simulink model "updated_target_driver_2026_withVariants"  (R2024b)
settings: Solver=FixedStepDiscrete  StartTime=0.0  StopTime=running_time  FixedStep=dt_s  RelTol=1e-3
values from neighbouring files (symbols this model uses):
  A = gamma_2*gamma_3*Thrust_desired    [force2voltage.m]
  a2_lb = -0.25    [target_driver_setup_2022_Ctrl_V_2_4.m]    (also in target_driver_setup_2022_Ctrl_V_2_4_geometric.m; target_driver_setup_mpc_12msdelay.m; target_driver_setup_mpc_andWLQP.m)
  a2_openloop = -0    (= 0)    [target_driver_setup_2022_Ctrl_V_2_4.m]    (also in target_driver_setup_2022_Ctrl_V_2_4_geometric.m = 0.6; target_driver_setup_mpc_12msdelay.m; target_driver_setup_mpc_andWLQP.m)
  a2_ub = 0.25    [target_driver_setup_2022_Ctrl_V_2_4.m]    (also in target_driver_setup_2022_Ctrl_V_2_4_geometric.m; target_driver_setup_mpc_12msdelay.m; target_driver_setup_mpc_andWLQP.m)
  adaptive_flag = 0    [target_driver_setup_2022_Ctrl_V_2_4.m]    (also in target_driver_setup_2022_Ctrl_V_2_4_geometric.m; target_driver_setup_mpc_12msdelay.m = 1; target_driver_setup_mpc_andWLQP.m = 1)
  adaptive_gain = [gamma_adaptive, adaptive_roll_limit, adaptive_pitch_limit, adaptive_yaw_limit, c_2_adaptive, gamma_lateral_adaptive, adaptive_x_limit, adaptive_y_limit, adaptive_z_limit, c_1_adaptive]    [target_driver_setup_2022_Ctrl_V_2_4.m]    (also in target_driver_setup_2022_Ctrl_V_2_4_geometric.m; target_driver_setup_mpc_12msdelay.m; target_driver_setup_mpc_andWLQP.m)
  adaptive_lateral_flag = 0    [target_driver_setup_2022_Ctrl_V_2_4.m]    (also in target_driver_setup_2022_Ctrl_V_2_4_geometric.m; target_driver_setup_mpc_12msdelay.m = 1; target_driver_setup_mpc_andWLQP.m = 1)
  adaptive_pitch_init = 0    [target_driver_setup_2022_Ctrl_V_2_4.m]    (also in target_driver_setup_2022_Ctrl_V_2_4_geometric.m; target_driver_setup_mpc_12msdelay.m; target_driver_setup_mpc_andWLQP.m)
  adaptive_pitch_limit = 0.1/(scale^2)    (= 1e-07)    [target_driver_setup_2022_Ctrl_V_2_4.m]    (also in target_driver_setup_2022_Ctrl_V_2_4_geometric.m = 3e-07; target_driver_setup_mpc_12msdelay.m; target_driver_setup_mpc_andWLQP.m)
  adaptive_pitch_limit_low = -adaptive_pitch_limit    (= -1e-07)    [target_driver_setup_2022_Ctrl_V_2_4.m]    (also in target_driver_setup_2022_Ctrl_V_2_4_geometric.m = -3e-07; target_driver_setup_mpc_12msdelay.m; target_driver_setup_mpc_andWLQP.m)
  adaptive_roll_init = 0    [target_driver_setup_2022_Ctrl_V_2_4.m]    (also in target_driver_setup_2022_Ctrl_V_2_4_geometric.m; target_driver_setup_mpc_12msdelay.m; target_driver_setup_mpc_andWLQP.m)
  adaptive_roll_limit = 0.3/(scale^2)    (= 3e-07)    [target_driver_setup_2022_Ctrl_V_2_4.m]    (also in target_driver_setup_2022_Ctrl_V_2_4_geometric.m; target_driver_setup_mpc_12msdelay.m; target_driver_setup_mpc_andWLQP.m)
  adaptive_roll_limit_low = -adaptive_roll_limit    (= -3e-07)    [target_driver_setup_2022_Ctrl_V_2_4.m]    (also in target_driver_setup_2022_Ctrl_V_2_4_geometric.m; target_driver_setup_mpc_12msdelay.m; target_driver_setup_mpc_andWLQP.m)
  adaptive_x_init = 0    [target_driver_setup_2022_Ctrl_V_2_4.m]    (also in target_driver_setup_2022_Ctrl_V_2_4_geometric.m; target_driver_setup_mpc_12msdelay.m; target_driver_setup_mpc_andWLQP.m)
  adaptive_x_limit = 0.15/(scale)    (= 0.00015)    [target_driver_setup_2022_Ctrl_V_2_4.m]    (also in target_driver_setup_2022_Ctrl_V_2_4_geometric.m = 7.5e-05; target_driver_setup_mpc_12msdelay.m; target_driver_setup_mpc_andWLQP.m)
  adaptive_x_limit_low = -adaptive_x_limit    (= -0.00015)    [target_driver_setup_2022_Ctrl_V_2_4.m]    (also in target_driver_setup_2022_Ctrl_V_2_4_geometric.m = -7.5e-05; target_driver_setup_mpc_12msdelay.m; target_driver_setup_mpc_andWLQP.m)
  adaptive_y_init = 0    [target_driver_setup_2022_Ctrl_V_2_4.m]    (also in target_driver_setup_2022_Ctrl_V_2_4_geometric.m; target_driver_setup_mpc_12msdelay.m; target_driver_setup_mpc_andWLQP.m)
  adaptive_y_limit = 0.15/(scale)    (= 0.00015)    [target_driver_setup_2022_Ctrl_V_2_4.m]    (also in target_driver_setup_2022_Ctrl_V_2_4_geometric.m = 7.5e-05; target_driver_setup_mpc_12msdelay.m; target_driver_setup_mpc_andWLQP.m)
  adaptive_y_limit_low = -adaptive_y_limit    (= -0.00015)    [target_driver_setup_2022_Ctrl_V_2_4.m]    (also in target_driver_setup_2022_Ctrl_V_2_4_geometric.m = -7.5e-05; target_driver_setup_mpc_12msdelay.m; target_driver_setup_mpc_andWLQP.m)
  adaptive_yaw_init = 0    [target_driver_setup_2022_Ctrl_V_2_4.m]    (also in target_driver_setup_2022_Ctrl_V_2_4_geometric.m; target_driver_setup_mpc_12msdelay.m; target_driver_setup_mpc_andWLQP.m)
  adaptive_yaw_limit = 0.035/(scale^2)    (= 3.5e-08)    [target_driver_setup_2022_Ctrl_V_2_4.m]    (also in target_driver_setup_2022_Ctrl_V_2_4_geometric.m; target_driver_setup_mpc_12msdelay.m; target_driver_setup_mpc_andWLQP.m)
  adaptive_yaw_limit_low = -adaptive_yaw_limit    (= -3.5e-08)    [target_driver_setup_2022_Ctrl_V_2_4.m]    (also in target_driver_setup_2022_Ctrl_V_2_4_geometric.m; target_driver_setup_mpc_12msdelay.m; target_driver_setup_mpc_andWLQP.m)
  adaptive_z_init = 0/scale    (= 0)    [target_driver_setup_2022_Ctrl_V_2_4.m]    (also in target_driver_setup_2022_Ctrl_V_2_4_geometric.m; target_driver_setup_mpc_12msdelay.m; target_driver_setup_mpc_andWLQP.m)
  adaptive_z_limit = 0.20/(scale)    (= 0.0002)    [target_driver_setup_2022_Ctrl_V_2_4.m]    (also in target_driver_setup_2022_Ctrl_V_2_4_geometric.m = 0.0008; target_driver_setup_mpc_12msdelay.m = 0.0008; target_driver_setup_mpc_andWLQP.m = 0.0008)
  adaptive_z_limit_low = -adaptive_z_limit/1    (= -0.0002)    [target_driver_setup_2022_Ctrl_V_2_4.m]    (also in target_driver_setup_2022_Ctrl_V_2_4_geometric.m = -0.0008; target_driver_setup_mpc_12msdelay.m = -0.0008; target_driver_setup_mpc_andWLQP.m = -0.0008)
  att_s = 500    [target_driver_setup_2022_Ctrl_V_2_4.m]    (also in target_driver_setup_2022_Ctrl_V_2_4_geometric.m; target_driver_setup_mpc_12msdelay.m; target_driver_setup_mpc_andWLQP.m)
  b_1_d_desired = [1,0,0]    [target_driver_setup_2022_Ctrl_V_2_4.m]    (also in target_driver_setup_2022_Ctrl_V_2_4_geometric.m; target_driver_setup_mpc_12msdelay.m; target_driver_setup_mpc_andWLQP.m)
  closedloop_flag = 1    [target_driver_setup_2022_Ctrl_V_2_4.m]    (also in target_driver_setup_2022_Ctrl_V_2_4_geometric.m = 0; target_driver_setup_mpc_12msdelay.m = 0; target_driver_setup_mpc_andWLQP.m = 0)
  control_gain = [k_x,k_v, k_R, k_Omega, k_z, k_vz, k_Rx]    [target_driver_setup_2022_Ctrl_V_2_4.m]    (also in target_driver_setup_2022_Ctrl_V_2_4_geometric.m = [k_x,k_v,k_R,k_Omega_pitch,k_Omega_roll,k_z,k_vz,k_Rx]; target_driver_setup_mpc_12msdelay.m = [k_x, k_v, k_R, k_Omega, k_z, k_vz, k_Rx,                  k; target_driver_setup_mpc_andWLQP.m = [k_x, k_v, k_R, k_Omega, k_z, k_vz, k_Rx,                  k)
  delay = delay-vicon_sample_cycle/2    [target_driver_setup_2022_Ctrl_V_2_4.m]    (also in target_driver_setup_2022_Ctrl_V_2_4_geometric.m; target_driver_setup_mpc_12msdelay.m; target_driver_setup_mpc_andWLQP.m)
  drv_amp = abs((vleft_p2p-vright_p2p))/2+min(vleft_p2p,vright_p2p)    [Wing_traj_to_Voltage.m]    (also in force2voltage.m; target_driver_setup_2022_Ctrl_V_2_4.m = 300; target_driver_setup_2022_Ctrl_V_2_4_geometric.m = 110; target_driver_setup_mpc_12msdelay.m = 150)
  drv_bias = max_drv_bias    (= 300)    [target_driver_setup_2022_Ctrl_V_2_4.m]    (also in target_driver_setup_2022_Ctrl_V_2_4_geometric.m = 200; target_driver_setup_mpc_12msdelay.m = 200; target_driver_setup_mpc_andWLQP.m = 200)
  drv_pitch_left = vleft_pitch    [Wing_traj_to_Voltage.m]    (also in force2voltage.m = 0; target_driver_setup_2022_Ctrl_V_2_4.m = 0; target_driver_setup_2022_Ctrl_V_2_4_geometric.m = 9.05; target_driver_setup_mpc_12msdelay.m = 9.05)
  drv_pitch_right = vright_pitch    [Wing_traj_to_Voltage.m]    (also in force2voltage.m = 0; target_driver_setup_2022_Ctrl_V_2_4.m = 0; target_driver_setup_2022_Ctrl_V_2_4_geometric.m = 9.05; target_driver_setup_mpc_12msdelay.m = 9.05)
  drv_roll = (vleft_p2p-vright_p2p)/4    [Wing_traj_to_Voltage.m]    (also in force2voltage.m; target_driver_setup_2022_Ctrl_V_2_4.m = 0; target_driver_setup_2022_Ctrl_V_2_4_geometric.m = -0.001; target_driver_setup_mpc_12msdelay.m = -0.001)
  dt_s = 1e-3    (= 0.001)    [target_driver_setup_2022_Ctrl_V_2_4.m]    (also in target_driver_setup_2022_Ctrl_V_2_4_geometric.m = 0.0002; target_driver_setup_mpc_12msdelay.m = 0.0002; target_driver_setup_mpc_andWLQP.m = 0.0002)
  f_fin = f    (= 180)    [target_driver_setup_2022_Ctrl_V_2_4.m]    (also in target_driver_setup_2022_Ctrl_V_2_4_geometric.m = 155; target_driver_setup_mpc_12msdelay.m = 155; target_driver_setup_mpc_andWLQP.m = 155)
  f_int = f    (= 180)    [target_driver_setup_2022_Ctrl_V_2_4.m]    (also in target_driver_setup_2022_Ctrl_V_2_4_geometric.m = 155; target_driver_setup_mpc_12msdelay.m = 155; target_driver_setup_mpc_andWLQP.m = 155)
  g = 9.8    [target_driver_setup_2022_Ctrl_V_2_4.m]    (also in target_driver_setup_2022_Ctrl_V_2_4_geometric.m; target_driver_setup_mpc_12msdelay.m; target_driver_setup_mpc_andWLQP.m = 9.81; test_full_attitude_mpc.m = 9.81)
  I_moment_vec = [Ixx, Iyy, Izz]    [target_driver_setup_2022_Ctrl_V_2_4.m]    (also in target_driver_setup_2022_Ctrl_V_2_4_geometric.m; target_driver_setup_mpc_12msdelay.m; target_driver_setup_mpc_andWLQP.m)
  landing_flag = 0    [target_driver_setup_2022_Ctrl_V_2_4.m]    (also in target_driver_setup_2022_Ctrl_V_2_4_geometric.m; target_driver_setup_mpc_12msdelay.m; target_driver_setup_mpc_andWLQP.m)
  landing_parameter = [start_delay+T,transition_rate, rising_time, falling_time, landing_rising_time, landing_z_decrease, landing_y_decrease, landing_x_decrease]    [target_driver_setup_2022_Ctrl_V_2_4.m]    (also in target_driver_setup_2022_Ctrl_V_2_4_geometric.m; target_driver_setup_mpc_12msdelay.m; target_driver_setup_mpc_andWLQP.m)
  low_bound = -8    [target_driver_setup_2022_Ctrl_V_2_4.m]    (also in target_driver_setup_2022_Ctrl_V_2_4_geometric.m = -5; target_driver_setup_mpc_12msdelay.m = -10; target_driver_setup_mpc_andWLQP.m = -10)
  low_bound_eR = -0.8    [target_driver_setup_2022_Ctrl_V_2_4.m]    (also in target_driver_setup_2022_Ctrl_V_2_4_geometric.m = -1.2; target_driver_setup_mpc_12msdelay.m = -1.2; target_driver_setup_mpc_andWLQP.m = -1.2)
  low_bound_vx = -0.5    [target_driver_setup_2022_Ctrl_V_2_4.m]    (also in target_driver_setup_2022_Ctrl_V_2_4_geometric.m; target_driver_setup_mpc_12msdelay.m; target_driver_setup_mpc_andWLQP.m)
  low_bound_vy = -0.5    [target_driver_setup_2022_Ctrl_V_2_4.m]    (also in target_driver_setup_2022_Ctrl_V_2_4_geometric.m; target_driver_setup_mpc_12msdelay.m; target_driver_setup_mpc_andWLQP.m)
  low_bound_vz = -0.5    [target_driver_setup_2022_Ctrl_V_2_4.m]    (also in target_driver_setup_2022_Ctrl_V_2_4_geometric.m; target_driver_setup_mpc_12msdelay.m; target_driver_setup_mpc_andWLQP.m)
  low_bound_x = -0.06    [target_driver_setup_2022_Ctrl_V_2_4.m]    (also in target_driver_setup_2022_Ctrl_V_2_4_geometric.m = -0.1; target_driver_setup_mpc_12msdelay.m = -0.6; target_driver_setup_mpc_andWLQP.m = -0.6)
  low_bound_y = -0.06    [target_driver_setup_2022_Ctrl_V_2_4.m]    (also in target_driver_setup_2022_Ctrl_V_2_4_geometric.m; target_driver_setup_mpc_12msdelay.m = -0.6; target_driver_setup_mpc_andWLQP.m = -0.6)
  low_bound_z = -0.04    [target_driver_setup_2022_Ctrl_V_2_4.m]    (also in target_driver_setup_2022_Ctrl_V_2_4_geometric.m; target_driver_setup_mpc_12msdelay.m = -0.1; target_driver_setup_mpc_andWLQP.m = -0.1)
  m = t <= t_zoom    [plot_roll_torque_cmd_vs_actual.m]    (also in plot_roll_torque_cmd_vs_actual_flightlog.m = t >= t0 & t <= t1; target_driver_setup_2022_Ctrl_V_2_4.m = 0.000124; target_driver_setup_2022_Ctrl_V_2_4_geometric.m = 8.5655e-05; target_driver_setup_mpc_12msdelay.m = 8.5655e-05)
  params_vec = [params_opt.delta_1, params_opt.delta_2, params_opt.delta_3,      params_opt.gamma_1, params_opt.gamma_2_1, params_opt.gamma_3,      params_opt.eta, params_opt.nu, params_opt.mu]'    [force2voltage_tuningSandbox.m]    (also in target_driver_setup_2022_Ctrl_V_2_4.m = [params_opt.delta_1, params_opt.delta_2, params_opt.delta_3,; target_driver_setup_2022_Ctrl_V_2_4_geometric.m = [params_opt.delta_1, params_opt.delta_2, params_opt.delta_3,; target_driver_setup_mpc_12msdelay.m = [params_opt.delta_1, params_opt.delta_2, params_opt.delta_3,; target_driver_setup_mpc_andWLQP.m = [params_opt.delta_1, params_opt.delta_2, params_opt.delta_3,)
  phase = 0    [target_driver_setup_2022_Ctrl_V_2_4.m]    (also in target_driver_setup_2022_Ctrl_V_2_4_geometric.m; target_driver_setup_mpc_12msdelay.m; target_driver_setup_mpc_andWLQP.m)
  r_desired = [default_x, default_y,z_desired]    [target_driver_setup_2022_Ctrl_V_2_4.m]    (also in target_driver_setup_2022_Ctrl_V_2_4_geometric.m; target_driver_setup_mpc_12msdelay.m; target_driver_setup_mpc_andWLQP.m)
  roll_offset_angle = 0    [target_driver_setup_2022_Ctrl_V_2_4.m]    (also in target_driver_setup_2022_Ctrl_V_2_4_geometric.m; target_driver_setup_mpc_12msdelay.m; target_driver_setup_mpc_andWLQP.m)
  running_time = start_delay+total_T    (= 9)    [target_driver_setup_2022_Ctrl_V_2_4.m]    (also in target_driver_setup_2022_Ctrl_V_2_4_geometric.m = 10; target_driver_setup_mpc_12msdelay.m = 0.5; target_driver_setup_mpc_andWLQP.m = 10)
  running_time_control = start_delay_control+total_T+0.0    (= 7.1)    [target_driver_setup_2022_Ctrl_V_2_4.m]    (also in target_driver_setup_2022_Ctrl_V_2_4_geometric.m = 10; target_driver_setup_mpc_12msdelay.m = 0.5; target_driver_setup_mpc_andWLQP.m = 10)
  sampling_f = 10000    [target_driver_setup_2022_Ctrl_V_2_4.m]    (also in target_driver_setup_2022_Ctrl_V_2_4_geometric.m = 5000; target_driver_setup_mpc_12msdelay.m = 5000; target_driver_setup_mpc_andWLQP.m = 5000)
  start_delay = 2.0    (= 2)    [target_driver_setup_2022_Ctrl_V_2_4.m]    (also in target_driver_setup_2022_Ctrl_V_2_4_geometric.m = 0; target_driver_setup_mpc_12msdelay.m = 0; target_driver_setup_mpc_andWLQP.m = 0)
  start_delay_control = start_delay + ramp_delay    (= 0.1)    [target_driver_setup_2022_Ctrl_V_2_4.m]    (also in target_driver_setup_2022_Ctrl_V_2_4_geometric.m = 0; target_driver_setup_mpc_12msdelay.m = 0; target_driver_setup_mpc_andWLQP.m = 0)
  T = 1    [target_driver_setup_2022_Ctrl_V_2_4.m]    (also in target_driver_setup_2022_Ctrl_V_2_4_geometric.m = 10; target_driver_setup_mpc_12msdelay.m = 0.5; target_driver_setup_mpc_andWLQP.m = 10; test_full_attitude_mpc.m = T0 + nu(1))
  task_flag = 0    [target_driver_setup_2022_Ctrl_V_2_4.m]    (also in target_driver_setup_2022_Ctrl_V_2_4_geometric.m; target_driver_setup_mpc_12msdelay.m; target_driver_setup_mpc_andWLQP.m)
  task_parameter = [radius_ref, frequency_ref, radius_ratio, lissajous_ratio, lissajous_delta, lissajous_amplitude_ratio,z_radius_ratio]    [target_driver_setup_2022_Ctrl_V_2_4.m]    (also in target_driver_setup_2022_Ctrl_V_2_4_geometric.m; target_driver_setup_mpc_12msdelay.m; target_driver_setup_mpc_andWLQP.m)
  upp_bound = 8    [target_driver_setup_2022_Ctrl_V_2_4.m]    (also in target_driver_setup_2022_Ctrl_V_2_4_geometric.m = 5; target_driver_setup_mpc_12msdelay.m = 10; target_driver_setup_mpc_andWLQP.m = 10)
  upp_bound_eR = 0.8    [target_driver_setup_2022_Ctrl_V_2_4.m]    (also in target_driver_setup_2022_Ctrl_V_2_4_geometric.m = 1.2; target_driver_setup_mpc_12msdelay.m = 1.2; target_driver_setup_mpc_andWLQP.m = 1.2)
  upp_bound_vx = 0.5    [target_driver_setup_2022_Ctrl_V_2_4.m]    (also in target_driver_setup_2022_Ctrl_V_2_4_geometric.m; target_driver_setup_mpc_12msdelay.m; target_driver_setup_mpc_andWLQP.m)
  upp_bound_vy = 0.5    [target_driver_setup_2022_Ctrl_V_2_4.m]    (also in target_driver_setup_2022_Ctrl_V_2_4_geometric.m; target_driver_setup_mpc_12msdelay.m; target_driver_setup_mpc_andWLQP.m)
  upp_bound_vz = 0.5    [target_driver_setup_2022_Ctrl_V_2_4.m]    (also in target_driver_setup_2022_Ctrl_V_2_4_geometric.m; target_driver_setup_mpc_12msdelay.m; target_driver_setup_mpc_andWLQP.m)
  upp_bound_x = 0.06    [target_driver_setup_2022_Ctrl_V_2_4.m]    (also in target_driver_setup_2022_Ctrl_V_2_4_geometric.m = 0.1; target_driver_setup_mpc_12msdelay.m = 0.6; target_driver_setup_mpc_andWLQP.m = 0.6)
  upp_bound_y = 0.06    [target_driver_setup_2022_Ctrl_V_2_4.m]    (also in target_driver_setup_2022_Ctrl_V_2_4_geometric.m; target_driver_setup_mpc_12msdelay.m = 0.6; target_driver_setup_mpc_andWLQP.m = 0.6)
  upp_bound_z = 0.04    [target_driver_setup_2022_Ctrl_V_2_4.m]    (also in target_driver_setup_2022_Ctrl_V_2_4_geometric.m; target_driver_setup_mpc_12msdelay.m = 0.1; target_driver_setup_mpc_andWLQP.m = 0.1)
undefined symbols (not defined in the file or in its folder): Com1, DiscIntNeverNeededParam, dspblkCoreblockFVToolHelper, gcbh, left_mapping, left_mapping_F_to_Phi, lp_den, lp_num, none, right_mapping, right_mapping_F_to_Phi, vlp_den, vlp_num
libraries: simulink x20, xpcseriallib x2, xpcnilib x1, xpcutilitieslib x1
(part 4 of 6)

== system updated_target_driver_2026_withVariants/Vicon Post Processing1/Vicon Validity check/Variant Subsystem1/Simulation ==
  In1 : Inport
  Discrete Pulse Generator : DiscretePulseGenerator  Period=5  SampleTime=dt_s
  Terminator : Terminator
  Out1 : Outport
  wires:
  Discrete Pulse Generator/1 -> Out1/1
  In1/1 -> Terminator/1

== system updated_target_driver_2026_withVariants/Variant Subsystem/Experimental/signal generator a3/Bias_Signal/AveragedBias ==
  note: To avoid having signal "jump",
      | we want SMOOTH transitions
      | in frequency (i.e., a weighted sum
      | of current freq and freq some delta t ago)
  note: time constant = 0.002sec
  In1 : Inport
  Discrete Transfer Fcn : DiscreteTransferFcn  Numerator=[0.05]  Denominator=[1 -.95]
  Out1 : Outport
  wires:
  In1/1 -> Discrete Transfer Fcn/1
  Discrete Transfer Fcn/1 -> Out1/1

== system updated_target_driver_2026_withVariants/Variant Subsystem/Experimental/signal generator a3/Bias_Signal/SIgnalForRamp_binary ==
  note: Should output 1 or -1,
      | so signal ramps UP to 1
      | or DOWN to 0.
  In1 : Inport
  Add : Sum  Inputs=+-
  Compare To Zero : simulink/Logic and Bit Operations/Compare To Zero  relop=>  OutDataTypeStr=uint8  ZeroCross=off
  Constant : Constant
  Data Type Conversion : DataTypeConversion  OutDataTypeStr=double  SaturateOnIntegerOverflow=off  RndMeth=Floor
  Gain : Gain  Gain=2
  Out1 : Outport
  wires:
  In1/1 -> Compare To Zero/1
  Compare To Zero/1 -> Data Type Conversion/1
  Gain/1 -> Add/1
  Constant/1 -> Add/2
  Add/1 -> Out1/1
  Data Type Conversion/1 -> Gain/1

== system updated_target_driver_2026_withVariants/Variant Subsystem/Experimental/signal generator a3/Drive_Signal/AveragedAmp_filtered ==
  note: To avoid having signal "jump",
      | we want SMOOTH transitions
      | in frequency (i.e., a weighted sum
      | of current freq and freq some delta t ago)
  note: time constant 0.002sec
      | for 10kHz samping
  In1 : Inport
  Discrete Transfer Fcn : DiscreteTransferFcn  Numerator=[0.05]  Denominator=[1 -.95]
  Out1 : Outport
  wires:
  In1/1 -> Discrete Transfer Fcn/1
  Discrete Transfer Fcn/1 -> Out1/1

== system updated_target_driver_2026_withVariants/Variant Subsystem/Experimental/signal generator a3/Drive_Signal/AveragedOffset_filtered ==
  note: To avoid having signal "jump",
      | we want SMOOTH transitions
      | in frequency (i.e., a weighted sum
      | of current freq and freq some delta t ago)
  note: c
  note: time constant 0.02sec
      | for 10kHz samping
  In1 : Inport
  Discrete Transfer Fcn : DiscreteTransferFcn  Numerator=[0.05]  Denominator=[1 -.95]
  Out1 : Outport
  wires:
  In1/1 -> Discrete Transfer Fcn/1
  Discrete Transfer Fcn/1 -> Out1/1

== system updated_target_driver_2026_withVariants/Variant Subsystem/Experimental/signal generator a3/Drive_Signal/FlattenedSine1 ==
  freq : Inport
  phase : Inport  Port=2
  a2 : Inport  Port=3
  0.1 : Gain  Gain=0.1
  1.1 : Gain  Gain=1.1
  2f : Gain  Gain=2
  2pi : Gain  Gain=2*pi
  3f : Gain  Gain=3
  Add : Sum  Inputs=+++
  Add1 : Sum
  Amplitude Correction : Subsystem  Commented=on
  AveragedAmp_filtered : Subsystem
  Product : Product
  first harmonic : Trigonometry  OutputSignalType=real
  integrate(omega*t) : DiscreteIntegrator  SampleTime=-1  ICPrevOutput=DiscIntNeverNeededParam  ICPrevScaledInput=DiscIntNeverNeededParam
  second harmonic : Trigonometry  OutputSignalType=real
  third harmonic : Trigonometry  OutputSignalType=real
  split cycle signal : Outport
  wires:
  freq/1 -> 2pi/1
  2pi/1 -> integrate(omega*t)/1
  3f/1 -> third harmonic/1
  first harmonic/1 -> 1.1/1
  third harmonic/1 -> 0.1/1
  1.1/1 -> Add/1
  Add1/1 -> first harmonic/1, 2f/1, 3f/1
  integrate(omega*t)/1 -> Add1/1
  phase/1 -> Add1/2
  2f/1 -> second harmonic/1
  0.1/1 -> Add/2
  Product/1 -> Add/3
  second harmonic/1 -> Product/1
  Add/1 -> split cycle signal/1
  a2/1 -> AveragedAmp_filtered/1(In1)
  AveragedAmp_filtered/1(Out1) -> Product/2

== system updated_target_driver_2026_withVariants/Variant Subsystem/Experimental/signal generator a3/Drive_Signal/FlattenedSine_phase ==
  f : Inport
  phase : Inport  Port=2
  0.1 : Gain  Gain=0.1
  1.1 : Gain  Gain=1.1
  2pi : Gain  Gain=2*pi
  3f : Gain  Gain=3
  Add : Sum
  Sum : Sum  Inputs=|++
  first harmonic : Trigonometry  OutputSignalType=real
  integrate(omega*t) : DiscreteIntegrator  SampleTime=-1  ICPrevOutput=DiscIntNeverNeededParam  ICPrevScaledInput=DiscIntNeverNeededParam
  pi/180 : Gain  Gain=pi/180
  third harmonic : Trigonometry  OutputSignalType=real
  split cycle signal : Outport
  wires:
  f/1 -> 2pi/1
  2pi/1 -> integrate(omega*t)/1
  3f/1 -> third harmonic/1
  first harmonic/1 -> 1.1/1
  third harmonic/1 -> 0.1/1
  1.1/1 -> Add/1
  0.1/1 -> Add/2
  Add/1 -> split cycle signal/1
  Sum/1 -> first harmonic/1, 3f/1
  pi/180/1 -> Sum/2
  integrate(omega*t)/1 -> Sum/1
  phase/1 -> pi/180/1

== system updated_target_driver_2026_withVariants/Variant Subsystem/Experimental/signal generator a3/Drive_Signal/SignalForRamp_binary ==
  note: Should output 1 or -1,
      | so signal ramps UP to 1
      | or DOWN to 0.
  In1 : Inport
  Add : Sum  Inputs=+-
  Compare To Zero : simulink/Logic and Bit Operations/Compare To Zero  relop=>  OutDataTypeStr=uint8  ZeroCross=off
  Constant : Constant
  Data Type Conversion : DataTypeConversion  OutDataTypeStr=double  SaturateOnIntegerOverflow=off  RndMeth=Floor
  Gain : Gain  Gain=2
  Out1 : Outport
  wires:
  In1/1 -> Compare To Zero/1
  Compare To Zero/1 -> Data Type Conversion/1
  Gain/1 -> Add/1
  Constant/1 -> Add/2
  Add/1 -> Out1/1
  Data Type Conversion/1 -> Gain/1

== system updated_target_driver_2026_withVariants/Variant Subsystem/Experimental/signal generator a3/Drive_Signal/SignalForSin_binary ==
  note: We want this to stay "high" for 1
      | second after the actual "enable"
      | is turned off...
  In1 : Inport
  Compare To Zero : simulink/Logic and Bit Operations/Compare To Zero  relop=>  OutDataTypeStr=uint8  ZeroCross=off
  Data Type Conversion : DataTypeConversion  OutDataTypeStr=double  SaturateOnIntegerOverflow=off  RndMeth=Floor
  Out1 : Outport
  wires:
  In1/1 -> Compare To Zero/1
  Compare To Zero/1 -> Data Type Conversion/1
  Data Type Conversion/1 -> Out1/1

== system updated_target_driver_2026_withVariants/Variant Subsystem/Experimental/signal generator a3/Drive_Signal/Sinewave ==
  In2 : Inport
  2pi : Gain  Gain=2*pi
  first harmonic : Trigonometry  OutputSignalType=real
  integrate(omega*t) : DiscreteIntegrator  SampleTime=-1  ICPrevOutput=DiscIntNeverNeededParam  ICPrevScaledInput=DiscIntNeverNeededParam
  split cycle signal : Outport
  wires:
  In2/1 -> 2pi/1
  2pi/1 -> integrate(omega*t)/1
  integrate(omega*t)/1 -> first harmonic/1
  first harmonic/1 -> split cycle signal/1

== system updated_target_driver_2026_withVariants/Variant Subsystem/Experimental/signal generator a3/Drive_Signal1/AveragedAmp_filtered ==
  note: To avoid having signal "jump",
      | we want SMOOTH transitions
      | in frequency (i.e., a weighted sum
      | of current freq and freq some delta t ago)
  note: time constant 0.002sec
      | for 10kHz samping
  In1 : Inport
  Discrete Transfer Fcn : DiscreteTransferFcn  Numerator=[0.05]  Denominator=[1 -.95]
  Out1 : Outport
  wires:
  In1/1 -> Discrete Transfer Fcn/1
  Discrete Transfer Fcn/1 -> Out1/1

== system updated_target_driver_2026_withVariants/Variant Subsystem/Experimental/signal generator a3/Drive_Signal1/AveragedOffset_filtered ==
  note: To avoid having signal "jump",
      | we want SMOOTH transitions
      | in frequency (i.e., a weighted sum
      | of current freq and freq some delta t ago)
  note: c
  note: time constant 0.02sec
      | for 10kHz samping
  In1 : Inport
  Discrete Transfer Fcn : DiscreteTransferFcn  LoadFcn=dspblkCoreblockFVToolHelper(gcbh,'load');  Numerator=[0.05]  Denominator=[1 -.95]
      settings: CopyFcn=dspblkCoreblockFVToolHelper(gcbh,'copy');  DeleteFcn=dspblkCoreblockFVToolHelper(gcbh,'close');  ModelCloseFcn=dspblkCoreblockFVToolHelper(gcbh,'close');  PreSaveFcn=dspblkCoreblockFVToolHelper(gcbh,'presave');  PostSaveFcn=dspblkCoreblockFVToolHelper(gcbh,'postsave');  CloseFcn=dspblkCoreblockFVToolHelper(gcbh,'close');
  Out1 : Outport
  wires:
  In1/1 -> Discrete Transfer Fcn/1
  Discrete Transfer Fcn/1 -> Out1/1

== system updated_target_driver_2026_withVariants/Variant Subsystem/Experimental/signal generator a3/Drive_Signal1/FlattenedSine1 ==
  freq : Inport
  a2 : Inport  Port=2
  0.1 : Gain  Gain=0.1
  0.2 : Gain  Gain=-1
  1.1 : Gain  Gain=1.1
  2f : Gain  Gain=2
  2pi : Gain  Gain=2*pi
  3f : Gain  Gain=3
  Add : Sum  Inputs=+++
  Amplitude Correction : Subsystem  Commented=on
  AveragedAmp_filtered : Subsystem
  Product : Product
  first harmonic : Trigonometry  OutputSignalType=real
  integrate(omega*t) : DiscreteIntegrator  SampleTime=-1  ICPrevOutput=DiscIntNeverNeededParam  ICPrevScaledInput=DiscIntNeverNeededParam
  second harmonic : Trigonometry  OutputSignalType=real
  third harmonic : Trigonometry  OutputSignalType=real
  split cycle signal : Outport
  wires:
  freq/1 -> 2pi/1
  2pi/1 -> integrate(omega*t)/1
  3f/1 -> third harmonic/1
  first harmonic/1 -> 1.1/1
  third harmonic/1 -> 0.1/1
  1.1/1 -> Add/1
  integrate(omega*t)/1 -> first harmonic/1, 2f/1, 3f/1
  2f/1 -> second harmonic/1
  0.1/1 -> Add/2
  Product/1 -> Add/3
  second harmonic/1 -> Product/1
  0.2/1 -> Product/2
  Add/1 -> split cycle signal/1
  a2/1 -> AveragedAmp_filtered/1(In1)
  AveragedAmp_filtered/1(Out1) -> 0.2/1

== system updated_target_driver_2026_withVariants/Variant Subsystem/Experimental/signal generator a3/Drive_Signal1/SignalForRamp_binary ==
  note: Should output 1 or -1,
      | so signal ramps UP to 1
      | or DOWN to 0.
  In1 : Inport
  Add : Sum  Inputs=+-
  Compare To Zero : simulink/Logic and Bit Operations/Compare To Zero  relop=>  OutDataTypeStr=uint8  ZeroCross=off
  Constant : Constant
  Data Type Conversion : DataTypeConversion  OutDataTypeStr=double  SaturateOnIntegerOverflow=off  RndMeth=Floor
  Gain : Gain  Gain=2
  Out1 : Outport
  wires:
  In1/1 -> Compare To Zero/1
  Compare To Zero/1 -> Data Type Conversion/1
  Gain/1 -> Add/1
  Constant/1 -> Add/2
  Add/1 -> Out1/1
  Data Type Conversion/1 -> Gain/1

== system updated_target_driver_2026_withVariants/Variant Subsystem/Experimental/signal generator a3/Drive_Signal1/SignalForSin_binary ==
  note: We want this to stay "high" for 1
      | second after the actual "enable"
      | is turned off...
  In1 : Inport
  Compare To Zero : simulink/Logic and Bit Operations/Compare To Zero  relop=>  OutDataTypeStr=uint8  ZeroCross=off
  Data Type Conversion : DataTypeConversion  OutDataTypeStr=double  SaturateOnIntegerOverflow=off  RndMeth=Floor
  Out1 : Outport
  wires:
  In1/1 -> Compare To Zero/1
  Compare To Zero/1 -> Data Type Conversion/1
  Data Type Conversion/1 -> Out1/1

== system updated_target_driver_2026_withVariants/Variant Subsystem/Experimental/signal generator a3/Drive_Signal1/Sine Wave ==
  In2 : Inport
  2pi : Gain  Gain=2*pi
  first harmonic : Trigonometry  OutputSignalType=real
  integrate(omega*t) : DiscreteIntegrator  SampleTime=-1  ICPrevOutput=DiscIntNeverNeededParam  ICPrevScaledInput=DiscIntNeverNeededParam
  split cycle signal : Outport
  wires:
  In2/1 -> 2pi/1
  2pi/1 -> integrate(omega*t)/1
  integrate(omega*t)/1 -> first harmonic/1
  first harmonic/1 -> split cycle signal/1

== system updated_target_driver_2026_withVariants/Variant Subsystem/Simulation/signal generator a3/Bias_Signal/AveragedBias ==
  note: To avoid having signal "jump",
      | we want SMOOTH transitions
      | in frequency (i.e., a weighted sum
      | of current freq and freq some delta t ago)
  note: time constant = 0.002sec
  In1 : Inport
  Discrete Transfer Fcn : DiscreteTransferFcn  LoadFcn=dspblkCoreblockFVToolHelper(gcbh,'load');  Numerator=[0.05]  Denominator=[1 -.95]
      settings: CopyFcn=dspblkCoreblockFVToolHelper(gcbh,'copy');  DeleteFcn=dspblkCoreblockFVToolHelper(gcbh,'close');  ModelCloseFcn=dspblkCoreblockFVToolHelper(gcbh,'close');  PreSaveFcn=dspblkCoreblockFVToolHelper(gcbh,'presave');  PostSaveFcn=dspblkCoreblockFVToolHelper(gcbh,'postsave');  CloseFcn=dspblkCoreblockFVToolHelper(gcbh,'close');
  Out1 : Outport
  wires:
  In1/1 -> Discrete Transfer Fcn/1
  Discrete Transfer Fcn/1 -> Out1/1

== system updated_target_driver_2026_withVariants/Variant Subsystem/Simulation/signal generator a3/Bias_Signal/SIgnalForRamp_binary ==
  note: Should output 1 or -1,
      | so signal ramps UP to 1
      | or DOWN to 0.
  In1 : Inport
  Add : Sum  Inputs=+-
  Compare To Zero : simulink/Logic and Bit Operations/Compare To Zero  relop=>  OutDataTypeStr=uint8  ZeroCross=off
  Constant : Constant
  Data Type Conversion : DataTypeConversion  OutDataTypeStr=double  SaturateOnIntegerOverflow=off  RndMeth=Floor
  Gain : Gain  Gain=2
  Out1 : Outport
  wires:
  In1/1 -> Compare To Zero/1
  Compare To Zero/1 -> Data Type Conversion/1
  Gain/1 -> Add/1
  Constant/1 -> Add/2
  Add/1 -> Out1/1
  Data Type Conversion/1 -> Gain/1

== system updated_target_driver_2026_withVariants/Variant Subsystem/Simulation/signal generator a3/Drive_Signal/AveragedAmp_filtered ==
  note: To avoid having signal "jump",
      | we want SMOOTH transitions
      | in frequency (i.e., a weighted sum
      | of current freq and freq some delta t ago)
  note: time constant 0.002sec
      | for 10kHz samping
  In1 : Inport
  Discrete Transfer Fcn : DiscreteTransferFcn  LoadFcn=dspblkCoreblockFVToolHelper(gcbh,'load');  Numerator=[0.05]  Denominator=[1 -.95]
      settings: CopyFcn=dspblkCoreblockFVToolHelper(gcbh,'copy');  DeleteFcn=dspblkCoreblockFVToolHelper(gcbh,'close');  ModelCloseFcn=dspblkCoreblockFVToolHelper(gcbh,'close');  PreSaveFcn=dspblkCoreblockFVToolHelper(gcbh,'presave');  PostSaveFcn=dspblkCoreblockFVToolHelper(gcbh,'postsave');  CloseFcn=dspblkCoreblockFVToolHelper(gcbh,'close');
  Out1 : Outport
  wires:
  In1/1 -> Discrete Transfer Fcn/1
  Discrete Transfer Fcn/1 -> Out1/1

== system updated_target_driver_2026_withVariants/Variant Subsystem/Simulation/signal generator a3/Drive_Signal/AveragedOffset_filtered ==
  note: To avoid having signal "jump",
      | we want SMOOTH transitions
      | in frequency (i.e., a weighted sum
      | of current freq and freq some delta t ago)
  note: c
  note: time constant 0.02sec
      | for 10kHz samping
  In1 : Inport
  Discrete Transfer Fcn : DiscreteTransferFcn  Numerator=[0.05]  Denominator=[1 -.95]
  Out1 : Outport
  wires:
  In1/1 -> Discrete Transfer Fcn/1
  Discrete Transfer Fcn/1 -> Out1/1

== system updated_target_driver_2026_withVariants/Variant Subsystem/Simulation/signal generator a3/Drive_Signal/FlattenedSine1 ==
  freq : Inport
  phase : Inport  Port=2
  a2 : Inport  Port=3
  0.1 : Gain  Gain=0.1
  1.1 : Gain  Gain=1.1
  2f : Gain  Gain=2
  2pi : Gain  Gain=2*pi
  3f : Gain  Gain=3
  Add : Sum  Inputs=+++
  Add1 : Sum
  Amplitude Correction : Subsystem  Commented=on
  AveragedAmp_filtered : Subsystem
  Product : Product
  first harmonic : Trigonometry  OutputSignalType=real
  integrate(omega*t) : DiscreteIntegrator  SampleTime=-1  ICPrevOutput=DiscIntNeverNeededParam  ICPrevScaledInput=DiscIntNeverNeededParam
  second harmonic : Trigonometry  OutputSignalType=real
  third harmonic : Trigonometry  OutputSignalType=real
  split cycle signal : Outport
  wires:
  freq/1 -> 2pi/1
  2pi/1 -> integrate(omega*t)/1
  3f/1 -> third harmonic/1
  first harmonic/1 -> 1.1/1
  third harmonic/1 -> 0.1/1
  1.1/1 -> Add/1
  Add1/1 -> first harmonic/1, 2f/1, 3f/1
  integrate(omega*t)/1 -> Add1/1
  phase/1 -> Add1/2
  2f/1 -> second harmonic/1
  0.1/1 -> Add/2
  Product/1 -> Add/3
  second harmonic/1 -> Product/1
  Add/1 -> split cycle signal/1
  a2/1 -> AveragedAmp_filtered/1(In1)
  AveragedAmp_filtered/1(Out1) -> Product/2

== system updated_target_driver_2026_withVariants/Variant Subsystem/Simulation/signal generator a3/Drive_Signal/FlattenedSine_phase ==
  f : Inport
  phase : Inport  Port=2
  0.1 : Gain  Gain=0.1
  1.1 : Gain  Gain=1.1
  2pi : Gain  Gain=2*pi
  3f : Gain  Gain=3
  Add : Sum
  Sum : Sum  Inputs=|++
  first harmonic : Trigonometry  OutputSignalType=real
  integrate(omega*t) : DiscreteIntegrator  SampleTime=-1  ICPrevOutput=DiscIntNeverNeededParam  ICPrevScaledInput=DiscIntNeverNeededParam
  pi/180 : Gain  Gain=pi/180
  third harmonic : Trigonometry  OutputSignalType=real
  split cycle signal : Outport
  wires:
  f/1 -> 2pi/1
  2pi/1 -> integrate(omega*t)/1
  3f/1 -> third harmonic/1
  first harmonic/1 -> 1.1/1
  third harmonic/1 -> 0.1/1
  1.1/1 -> Add/1
  0.1/1 -> Add/2
  Add/1 -> split cycle signal/1
  Sum/1 -> first harmonic/1, 3f/1
  pi/180/1 -> Sum/2
  integrate(omega*t)/1 -> Sum/1
  phase/1 -> pi/180/1

== system updated_target_driver_2026_withVariants/Variant Subsystem/Simulation/signal generator a3/Drive_Signal/SignalForRamp_binary ==
  note: Should output 1 or -1,
      | so signal ramps UP to 1
      | or DOWN to 0.
  In1 : Inport
  Add : Sum  Inputs=+-
  Compare To Zero : simulink/Logic and Bit Operations/Compare To Zero  relop=>  OutDataTypeStr=uint8  ZeroCross=off
  Constant : Constant
  Data Type Conversion : DataTypeConversion  OutDataTypeStr=double  SaturateOnIntegerOverflow=off  RndMeth=Floor
  Gain : Gain  Gain=2
  Out1 : Outport
  wires:
  In1/1 -> Compare To Zero/1
  Compare To Zero/1 -> Data Type Conversion/1
  Gain/1 -> Add/1
  Constant/1 -> Add/2
  Add/1 -> Out1/1
  Data Type Conversion/1 -> Gain/1

== system updated_target_driver_2026_withVariants/Variant Subsystem/Simulation/signal generator a3/Drive_Signal/SignalForSin_binary ==
  note: We want this to stay "high" for 1
      | second after the actual "enable"
      | is turned off...
  In1 : Inport
  Compare To Zero : simulink/Logic and Bit Operations/Compare To Zero  relop=>  OutDataTypeStr=uint8  ZeroCross=off
  Data Type Conversion : DataTypeConversion  OutDataTypeStr=double  SaturateOnIntegerOverflow=off  RndMeth=Floor
  Out1 : Outport
  wires:
  In1/1 -> Compare To Zero/1
  Compare To Zero/1 -> Data Type Conversion/1
  Data Type Conversion/1 -> Out1/1

== system updated_target_driver_2026_withVariants/Variant Subsystem/Simulation/signal generator a3/Drive_Signal/Sinewave ==
  In2 : Inport
  2pi : Gain  Gain=2*pi
  first harmonic : Trigonometry  OutputSignalType=real
  integrate(omega*t) : DiscreteIntegrator  SampleTime=-1  ICPrevOutput=DiscIntNeverNeededParam  ICPrevScaledInput=DiscIntNeverNeededParam
  split cycle signal : Outport
  wires:
  In2/1 -> 2pi/1
  2pi/1 -> integrate(omega*t)/1
  integrate(omega*t)/1 -> first harmonic/1
  first harmonic/1 -> split cycle signal/1

== system updated_target_driver_2026_withVariants/Variant Subsystem/Simulation/signal generator a3/Drive_Signal1/AveragedAmp_filtered ==
  note: To avoid having signal "jump",
      | we want SMOOTH transitions
      | in frequency (i.e., a weighted sum
      | of current freq and freq some delta t ago)
  note: time constant 0.002sec
      | for 10kHz samping
  In1 : Inport
  Discrete Transfer Fcn1 : DiscreteTransferFcn  LoadFcn=dspblkCoreblockFVToolHelper(gcbh,'load');  Numerator=[0.05]  Denominator=[1 -.95]
      settings: CopyFcn=dspblkCoreblockFVToolHelper(gcbh,'copy');  DeleteFcn=dspblkCoreblockFVToolHelper(gcbh,'close');  ModelCloseFcn=dspblkCoreblockFVToolHelper(gcbh,'close');  PreSaveFcn=dspblkCoreblockFVToolHelper(gcbh,'presave');  PostSaveFcn=dspblkCoreblockFVToolHelper(gcbh,'postsave');  CloseFcn=dspblkCoreblockFVToolHelper(gcbh,'close');
  Out1 : Outport
  wires:
  In1/1 -> Discrete Transfer Fcn1/1
  Discrete Transfer Fcn1/1 -> Out1/1

== system updated_target_driver_2026_withVariants/Variant Subsystem/Simulation/signal generator a3/Drive_Signal1/AveragedOffset_filtered ==
  note: To avoid having signal "jump",
      | we want SMOOTH transitions
      | in frequency (i.e., a weighted sum
      | of current freq and freq some delta t ago)
  note: c
  note: time constant 0.02sec
      | for 10kHz samping
  In1 : Inport
  Discrete Transfer Fcn1 : DiscreteTransferFcn  LoadFcn=dspblkCoreblockFVToolHelper(gcbh,'load');  Numerator=[0.05]  Denominator=[1 -.95]
      settings: CopyFcn=dspblkCoreblockFVToolHelper(gcbh,'copy');  DeleteFcn=dspblkCoreblockFVToolHelper(gcbh,'close');  ModelCloseFcn=dspblkCoreblockFVToolHelper(gcbh,'close');  PreSaveFcn=dspblkCoreblockFVToolHelper(gcbh,'presave');  PostSaveFcn=dspblkCoreblockFVToolHelper(gcbh,'postsave');  CloseFcn=dspblkCoreblockFVToolHelper(gcbh,'close');
  Out1 : Outport
  wires:
  In1/1 -> Discrete Transfer Fcn1/1
  Discrete Transfer Fcn1/1 -> Out1/1

== system updated_target_driver_2026_withVariants/Variant Subsystem/Simulation/signal generator a3/Drive_Signal1/FlattenedSine1 ==
  freq : Inport
  a2 : Inport  Port=2
  0.1 : Gain  Gain=0.1
  0.2 : Gain  Gain=-1
  1.1 : Gain  Gain=1.1
  2f : Gain  Gain=2
  2pi : Gain  Gain=2*pi
  3f : Gain  Gain=3
  Add : Sum  Inputs=+++
  Amplitude Correction : Subsystem  Commented=on
  AveragedAmp_filtered : Subsystem
  Product : Product
  first harmonic : Trigonometry  OutputSignalType=real
  integrate(omega*t) : DiscreteIntegrator  SampleTime=-1  ICPrevOutput=DiscIntNeverNeededParam  ICPrevScaledInput=DiscIntNeverNeededParam
  second harmonic : Trigonometry  OutputSignalType=real
  third harmonic : Trigonometry  OutputSignalType=real
  split cycle signal : Outport
  wires:
  freq/1 -> 2pi/1
  2pi/1 -> integrate(omega*t)/1
  3f/1 -> third harmonic/1
  first harmonic/1 -> 1.1/1
  third harmonic/1 -> 0.1/1
  1.1/1 -> Add/1
  integrate(omega*t)/1 -> first harmonic/1, 2f/1, 3f/1
  2f/1 -> second harmonic/1
  0.1/1 -> Add/2
  Product/1 -> Add/3
  second harmonic/1 -> Product/1
  0.2/1 -> Product/2
  Add/1 -> split cycle signal/1
  a2/1 -> AveragedAmp_filtered/1(In1)
  AveragedAmp_filtered/1(Out1) -> 0.2/1

== system updated_target_driver_2026_withVariants/Variant Subsystem/Simulation/signal generator a3/Drive_Signal1/SignalForRamp_binary ==
  note: Should output 1 or -1,
      | so signal ramps UP to 1
      | or DOWN to 0.
  In1 : Inport
  Add : Sum  Inputs=+-
  Compare To Zero : simulink/Logic and Bit Operations/Compare To Zero  relop=>  OutDataTypeStr=uint8  ZeroCross=off
  Constant : Constant
  Data Type Conversion : DataTypeConversion  OutDataTypeStr=double  SaturateOnIntegerOverflow=off  RndMeth=Floor
  Gain : Gain  Gain=2
  Out1 : Outport
  wires:
  In1/1 -> Compare To Zero/1
  Compare To Zero/1 -> Data Type Conversion/1
  Gain/1 -> Add/1
  Constant/1 -> Add/2
  Add/1 -> Out1/1
  Data Type Conversion/1 -> Gain/1

== system updated_target_driver_2026_withVariants/Variant Subsystem/Simulation/signal generator a3/Drive_Signal1/SignalForSin_binary ==
  note: We want this to stay "high" for 1
      | second after the actual "enable"
      | is turned off...
  In1 : Inport
  Compare To Zero : simulink/Logic and Bit Operations/Compare To Zero  relop=>  OutDataTypeStr=uint8  ZeroCross=off
  Data Type Conversion : DataTypeConversion  OutDataTypeStr=double  SaturateOnIntegerOverflow=off  RndMeth=Floor
  Out1 : Outport
  wires:
  In1/1 -> Compare To Zero/1
  Compare To Zero/1 -> Data Type Conversion/1
  Data Type Conversion/1 -> Out1/1

== system updated_target_driver_2026_withVariants/Variant Subsystem/Simulation/signal generator a3/Drive_Signal1/Sine Wave ==
  In2 : Inport
  2pi : Gain  Gain=2*pi
  first harmonic : Trigonometry  OutputSignalType=real
  integrate(omega*t) : DiscreteIntegrator  SampleTime=-1  ICPrevOutput=DiscIntNeverNeededParam  ICPrevScaledInput=DiscIntNeverNeededParam
  split cycle signal : Outport
  wires:
  In2/1 -> 2pi/1
  2pi/1 -> integrate(omega*t)/1
  integrate(omega*t)/1 -> first harmonic/1
  first harmonic/1 -> split cycle signal/1

== system updated_target_driver_2026_withVariants/Variant Subsystem/Experimental/signal generator a3/Drive_Signal/FlattenedSine1/Amplitude Correction ==
  y : Inport
  a2 : Inport  Port=2
  Abs : Abs  SaturateOnIntegerOverflow=off
  Constant : Constant  Value=1.2
  Constant1 : Constant  Value=1.1
  Divide : Product  Inputs=*/
  Product1 : Product
  Sqrt : Sqrt
  Subtract : Sum  Inputs=+-
  y_new : Outport
  wires:
  Constant/1 -> Subtract/1
  Subtract/1 -> Sqrt/1
  Abs/1 -> Subtract/2
  a2/1 -> Abs/1
  y/1 -> Product1/1
  Product1/1 -> y_new/1
  Divide/1 -> Product1/2
  Constant1/1 -> Divide/2
  Sqrt/1 -> Divide/1

== system updated_target_driver_2026_withVariants/Variant Subsystem/Experimental/signal generator a3/Drive_Signal/FlattenedSine1/AveragedAmp_filtered ==
  note: To avoid having signal "jump",
      | we want SMOOTH transitions
      | in frequency (i.e., a weighted sum
      | of current freq and freq some delta t ago)
  note: time constant 0.002sec
      | for 10kHz samping
  In1 : Inport
  Discrete Transfer Fcn : DiscreteTransferFcn  Numerator=[0.05]  Denominator=[1 -.95]
  Out1 : Outport
  wires:
  In1/1 -> Discrete Transfer Fcn/1
  Discrete Transfer Fcn/1 -> Out1/1

== system updated_target_driver_2026_withVariants/Variant Subsystem/Experimental/signal generator a3/Drive_Signal1/FlattenedSine1/Amplitude Correction ==
  y : Inport
  a2 : Inport  Port=2
  Abs : Abs  SaturateOnIntegerOverflow=off
  Constant : Constant  Value=1.2
  Constant1 : Constant  Value=1.1
  Divide : Product  Inputs=*/
  Product1 : Product
  Sqrt : Sqrt
  Subtract : Sum  Inputs=+-
  y_new : Outport
  wires:
  Constant/1 -> Subtract/1
  Subtract/1 -> Sqrt/1
  Abs/1 -> Subtract/2
  a2/1 -> Abs/1
  y/1 -> Product1/1
  Product1/1 -> y_new/1
  Divide/1 -> Product1/2
  Constant1/1 -> Divide/2
  Sqrt/1 -> Divide/1

== system updated_target_driver_2026_withVariants/Variant Subsystem/Experimental/signal generator a3/Drive_Signal1/FlattenedSine1/AveragedAmp_filtered ==
  note: To avoid having signal "jump",
      | we want SMOOTH transitions
      | in frequency (i.e., a weighted sum
      | of current freq and freq some delta t ago)
  note: time constant 0.002sec
      | for 10kHz samping
  In1 : Inport
  Discrete Transfer Fcn : DiscreteTransferFcn  Numerator=[0.05]  Denominator=[1 -.95]
  Out1 : Outport
  wires:
  In1/1 -> Discrete Transfer Fcn/1
  Discrete Transfer Fcn/1 -> Out1/1

== system updated_target_driver_2026_withVariants/Variant Subsystem/Simulation/signal generator a3/Drive_Signal/FlattenedSine1/Amplitude Correction ==
  y : Inport
  a2 : Inport  Port=2
  Abs : Abs  SaturateOnIntegerOverflow=off
  Constant : Constant  Value=1.2
  Constant1 : Constant  Value=1.1
  Divide : Product  Inputs=*/
  Product1 : Product
  Sqrt : Sqrt
  Subtract : Sum  Inputs=+-
  y_new : Outport
  wires:
  Constant/1 -> Subtract/1
  Subtract/1 -> Sqrt/1
  Abs/1 -> Subtract/2
  a2/1 -> Abs/1
  y/1 -> Product1/1
  Product1/1 -> y_new/1
  Divide/1 -> Product1/2
  Constant1/1 -> Divide/2
  Sqrt/1 -> Divide/1

== system updated_target_driver_2026_withVariants/Variant Subsystem/Simulation/signal generator a3/Drive_Signal/FlattenedSine1/AveragedAmp_filtered ==
  note: To avoid having signal "jump",
      | we want SMOOTH transitions
      | in frequency (i.e., a weighted sum
      | of current freq and freq some delta t ago)
  note: time constant 0.002sec
      | for 10kHz samping
  In1 : Inport
  Discrete Transfer Fcn : DiscreteTransferFcn  Numerator=[0.05]  Denominator=[1 -.95]
  Out1 : Outport
  wires:
  In1/1 -> Discrete Transfer Fcn/1
  Discrete Transfer Fcn/1 -> Out1/1

== system updated_target_driver_2026_withVariants/Variant Subsystem/Simulation/signal generator a3/Drive_Signal1/FlattenedSine1/Amplitude Correction ==
  y : Inport
  a2 : Inport  Port=2
  Abs : Abs  SaturateOnIntegerOverflow=off
  Constant : Constant  Value=1.2
  Constant1 : Constant  Value=1.1
  Divide : Product  Inputs=*/
  Product1 : Product
  Sqrt : Sqrt
  Subtract : Sum  Inputs=+-
  y_new : Outport
  wires:
  Constant/1 -> Subtract/1
  Subtract/1 -> Sqrt/1
  Abs/1 -> Subtract/2
  a2/1 -> Abs/1
  y/1 -> Product1/1
  Product1/1 -> y_new/1
  Divide/1 -> Product1/2
  Constant1/1 -> Divide/2
  Sqrt/1 -> Divide/1

== system updated_target_driver_2026_withVariants/Variant Subsystem/Simulation/signal generator a3/Drive_Signal1/FlattenedSine1/AveragedAmp_filtered ==
  note: To avoid having signal "jump",
      | we want SMOOTH transitions
      | in frequency (i.e., a weighted sum
      | of current freq and freq some delta t ago)
  note: time constant 0.002sec
      | for 10kHz samping
  In1 : Inport
  Discrete Transfer Fcn : DiscreteTransferFcn  Numerator=[0.05]  Denominator=[1 -.95]
  Out1 : Outport
  wires:
  In1/1 -> Discrete Transfer Fcn/1
  Discrete Transfer Fcn/1 -> Out1/1

== matlab function updated_target_driver_2026_withVariants/Geometric Controller/lateral adaptive/Adaptive Control ==
  data: current_adaptive_x input; current_adaptive_y input; current_adaptive_z input; der_adaptive_torque_x output size=[1 1]; e_x input; e_v input; adaptive_gain_limit input; der_adaptive_torque_y output size=[1 1]; der_adaptive_torque_z output size=[1 1]
function [der_adaptive_torque_x, der_adaptive_torque_y, der_adaptive_torque_z] = fcn(current_adaptive_x,current_adaptive_y,current_adaptive_z, e_x,e_v,adaptive_gain_limit)


% Current state of adaptation
adaptive_torque_x=current_adaptive_x;
adaptive_torque_y=current_adaptive_y;
adaptive_torque_z=current_adaptive_z;

% Adaptive control parameters
gamma_lateral_adaptive = adaptive_gain_limit(6);
adaptvie_x_limit = adaptive_gain_limit(7);
adaptvie_y_limit = adaptive_gain_limit(8);
adaptvie_z_limit = adaptive_gain_limit(9);
c_1 = adaptive_gain_limit(10);

% Flag indicating the limit
adaptive_flag_x = adaptive_torque_x*(e_v(1)+c_1*e_x(1));
adaptive_flag_y = adaptive_torque_y*(e_v(2)+c_1*e_x(2));
adaptive_flag_z = adaptive_torque_z*(e_v(3)+c_1*e_x(3));

% size(adaptive_flag_x)

% derivative for desired adaptation
der_adaptive = gamma_lateral_adaptive*(e_v+c_1*e_x);

% epsillon=1e-15;


if (adaptive_flag_x<=0 && abs(adaptive_torque_x)==adaptvie_x_limit) || abs(adaptive_torque_x)<adaptvie_x_limit
	
	der_adaptive_torque_x=der_adaptive(1);
else
	der_adaptive_torque_x = 0;
end

if (adaptive_flag_y<=0 && abs(adaptive_torque_y)==adaptvie_y_limit) || abs(adaptive_torque_y)<adaptvie_y_limit
	
	der_adaptive_torque_y=der_adaptive(2);
else
	der_adaptive_torque_y = 0;
	
end

if (adaptive_flag_z<=0 && abs(adaptive_torque_z)==adaptvie_z_limit)|| abs(adaptive_torque_z)<adaptvie_z_limit
	
	der_adaptive_torque_z=der_adaptive(3);
else
	der_adaptive_torque_z = 0;
	
end


end

== matlab function updated_target_driver_2026_withVariants/Variant Subsystem/Simulation/Drake 2 Controller Axes1 ==
  data: x_drake input; x output; y_drake input; z_drake input; y output; z output
function [x,y,z] = fcn(x_drake,y_drake,z_drake)

    [x,y,z] = drake2controllerposition(x_drake,y_drake,z_drake); 

end

== matlab function updated_target_driver_2026_withVariants/Desired attitude and normalized error/Variant Subsystem/saturated normalized error observation/Saturated angular velocity eOmega /Compute attitude error eR ==
  data: y output size=[3 1]; R_cur input; R_desired input; omega input; omega_desired input
function y  = fcn(R_cur,R_desired,omega, omega_desired)

Rot_cur = [R_cur(1), R_cur(2), R_cur(3); R_cur(4), R_cur(5), R_cur(6); R_cur(7), R_cur(8), R_cur(9)];
Rot_desired = [R_desired(1), R_desired(2), R_desired(3); R_desired(4), R_desired(5), R_desired(6); R_desired(7), R_desired(8), R_desired(9)];
eOmega=zeros(3,1);
eOmega = omega - Rot_cur'*Rot_desired*omega_desired;

y = eOmega;

end

== matlab function updated_target_driver_2026_withVariants/Desired attitude and normalized error/Variant Subsystem/saturated normalized error observation/Saturated normalized eR/Compute attitude error eR ==
  data: y output size=[3 1]; R_cur input; R_desired input
function y  = fcn(R_cur,R_desired)

Rot_cur = [R_cur(1), R_cur(2), R_cur(3); R_cur(4), R_cur(5), R_cur(6); R_cur(7), R_cur(8), R_cur(9)];
Rot_desired = [R_desired(1), R_desired(2), R_desired(3); R_desired(4), R_desired(5), R_desired(6); R_desired(7), R_desired(8), R_desired(9)];
eR_so3=zeros(3,3);
eR_so3 = 1/2*(Rot_desired.'*Rot_cur-Rot_cur.'*Rot_desired);

eR = zeros(3,1);
eR(1) = eR_so3(3,2);
eR(2) = eR_so3(1,3);
eR(3) = eR_so3(2,1);

y = eR;

% Rot_desired 
end
